simulink model "aaa1"  (R2021b)
settings: Solver=VariableStepAuto  StartTime=0.0  StopTime=4  RelTol=1e-3
libraries: simulink x1
settings Model: Creator=郭义月  LastModifiedBy=郭义月

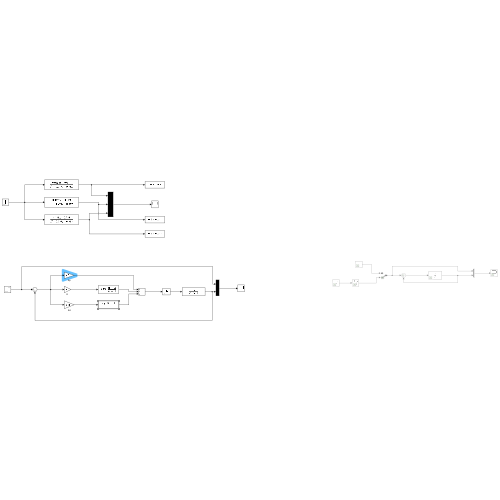
[thumbnail: Simulink's stored preview of the top-level diagram]
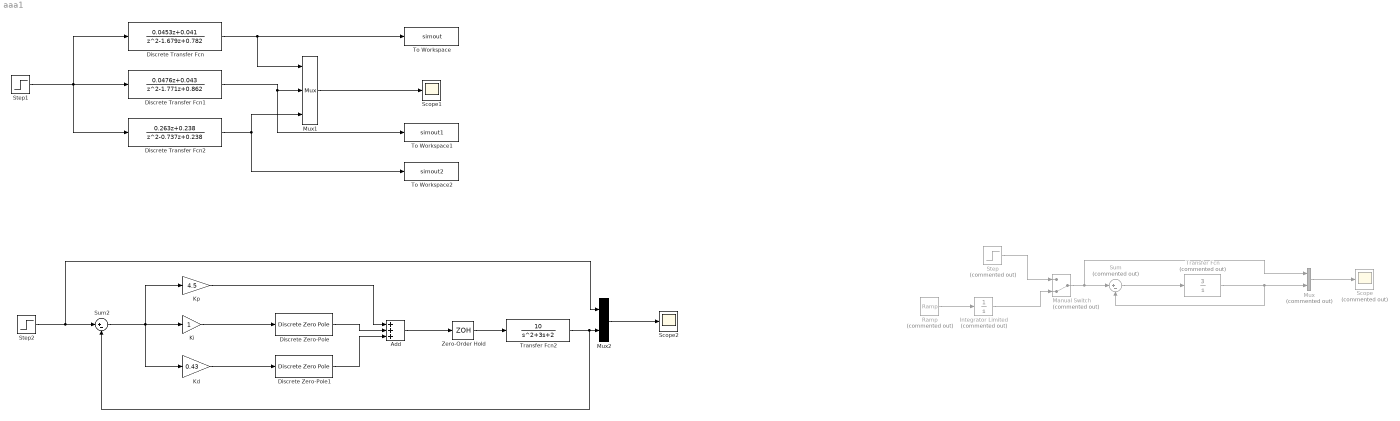
== system aaa1 ==
  Add : Sum  Inputs=+++
  Discrete Transfer Fcn : DiscreteTransferFcn  Numerator=[0.0453 0.041]  Denominator=[1 -1.679 0.782]
  Discrete Transfer Fcn1 : DiscreteTransferFcn  Numerator=[0.0476 0.043]  Denominator=[1 -1.771 0.862]
  Discrete Transfer Fcn2 : DiscreteTransferFcn  Numerator=[0.263 0.238]  Denominator=[1 -0.737 0.238]
  Discrete Zero-Pole : DiscreteZeroPole  Zeros=[-1]  Poles=[1]  Gain=0.05  SampleTime=-1
  Discrete Zero-Pole1 : DiscreteZeroPole  Poles=[0]  Gain=10  SampleTime=-1
  Integrator Limited : Integrator  Commented=on  LimitOutput=on  UpperSaturationLimit=1000  LowerSaturationLimit=0
  Kd : Gain  Gain=0.43
  Ki : Gain
  Kp : Gain  Gain=4.5
  Manual Switch : ManualSwitch  Commented=on  CurrentSetting=0
  Mux : Mux  Commented=on  Inputs=2
  Mux1 : Mux  Inputs=3
  Mux2 : Mux  Inputs=2
  Ramp : simulink/Sources/Ramp  Commented=on  slope=1  start=0  InitialOutput=0
  Scope : Scope  Commented=on
  Scope1 : Scope
  Scope2 : Scope
  Step : Step  Commented=on  SampleTime=0
  Step1 : Step  SampleTime=0
  Step2 : Step  SampleTime=0
  Sum : Sum  Commented=on  Inputs=|+-
  Sum2 : Sum  Inputs=|+-
  To Workspace : ToWorkspace  VariableName=simout  SaveFormat=Timeseries  SampleTime=-1
  To Workspace1 : ToWorkspace  VariableName=simout1  SaveFormat=Timeseries  SampleTime=-1
  To Workspace2 : ToWorkspace  VariableName=simout2  SaveFormat=Timeseries  SampleTime=-1
  Transfer Fcn : TransferFcn  Commented=on  Numerator=[3]  Denominator=[1 0]
  Transfer Fcn2 : TransferFcn  Numerator=[10]  Denominator=[1 3 2]
  Zero-Order Hold : ZeroOrderHold  SampleTime=-1
  wires:
  Step/1 -> Manual Switch/1
  Ramp/1 -> Integrator Limited/1
  Sum/1 -> Transfer Fcn/1
  Transfer Fcn/1 -> Mux/2, Sum/2
  Mux/1 -> Scope/1
  Manual Switch/1 -> Mux/1, Sum/1
  Integrator Limited/1 -> Manual Switch/2
  Mux2/1 -> Scope2/1
  Transfer Fcn2/1 -> Sum2/2, Mux2/2
  Step2/1 -> Mux2/1, Sum2/1
  Ki/1 -> Discrete Zero-Pole/1
  Kd/1 -> Discrete Zero-Pole1/1
  Discrete Zero-Pole/1 -> Add/2
  Discrete Zero-Pole1/1 -> Add/3
  Kp/1 -> Add/1
  Sum2/1 -> Kd/1, Ki/1, Kp/1
  Add/1 -> Zero-Order Hold/1
  Zero-Order Hold/1 -> Transfer Fcn2/1
  Step1/1 -> Discrete Transfer Fcn2/1, Discrete Transfer Fcn/1, Discrete Transfer Fcn1/1
  Discrete Transfer Fcn/1 -> Mux1/1, To Workspace/1
  Discrete Transfer Fcn1/1 -> To Workspace1/1, Mux1/2
  Discrete Transfer Fcn2/1 -> Mux1/3, To Workspace2/1
  Mux1/1 -> Scope1/1
